simulink model "stateflow_stateLanguage"  (R2015b)
settings: Solver=FixedStepDiscrete  StartTime=0.0  StopTime=10.0  RelTol=1e-3
settings Model: Creator=amyyang  LastModifiedBy=amyyang
settings OptimizationCC: DefaultParameterBehavior=Inlined  OptimizeModelRefInitCode=on  LifeSpan=1
settings RTWCC: SystemTargetFile=ert.tlc  GenCodeOnly=on  TemplateMakefile=ert_default_tmf  Description=Embedded Coder  GenerateReport=on  IncludeHyperlinkInReport=on  LaunchReport=on  GenerateTraceInfo=on  GenerateTraceReport=on  GenerateTraceReportSl=on  GenerateTraceReportSf=on  GenerateTraceReportEml=on
settings CodeAppCC: IgnoreCustomStorageClasses=off
settings ERTTargetCC: GenerateSampleERTMain=on  InlinedParameterPlacement=NonHierarchical  ERTCustomFileTemplate=example_file_process.tlc

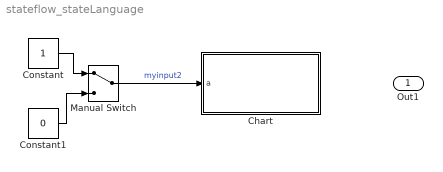
== system stateflow_stateLanguage ==
  Chart : Stateflow chart  TreatAsAtomicUnit=on
  Constant : Constant
  Constant1 : Constant  Value=0
  Manual Switch : ManualSwitch
  Out1 : Outport
  wires:
  ? -> Out1/1  "out2"
  Manual Switch/1 -> Chart/1(a)  "myinput2"
  Constant/1 -> Manual Switch/1
  Constant1/1 -> Manual Switch/2

== stateflow chart stateflow_stateLanguage/Chart ==
  state State3
    en:
    en_value = 1;
    en_value2 = 2;
    /* 注释不要断行 */
    // 断行用这种符号
  note: en,du,ex都另起一行；
      | 每一行执行语句后一定加分号，不然把结果打印到命令行影响仿真速度;
  note: en语句顶格
  note: 执行语句前面加个空格
  note: 条件语句前不要有空格
  note: 统一在二元运算符前后都加空格
      | 一元运算符不要加，比如b++
  note: 执行语句换行后，加空格
  state State4
    en:
    en_value = 1;
    en_value2 = 2;
    /* 这样断行写,注释就不清楚
    如果中间加入
    en_value2 = a;
    的解释语句的话 */
  note: 各种语句要布置美观，不要超出模块边界
  (default) -> State3
  State3 -> State4 : [a > 0]
      | {
      |  c = b;
      | }
  State4 -> State3 : [a < 1]
  data: a input
